simulink model "x_loop"  (Simulink 8.2)
settings: Solver=ode45  StartTime=0.0  StopTime=50  RelTol=1e-3
undefined symbols (not defined in the file): P
settings Model: Creator=paul  LastModifiedBy=paul
settings DataIOCC: SignalLoggingSaveFormat=Dataset
settings OptimizationCC: ExpressionDepthLimit=128
settings DebuggingCC: FcnCallInpInsideContextMsg=EnableAllAsError  StateNameClashWarn=none
settings GRTTargetCC: CombineOutputUpdateFcns=on  GRTInterface=off
settings ConfigurationSet: Description=SimMechanics 2G

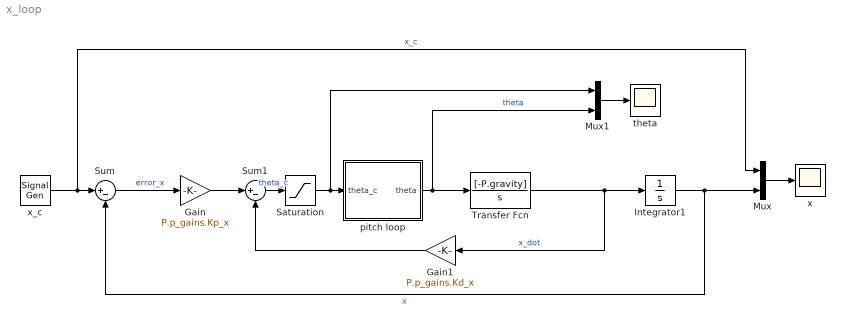
== system x_loop ==
  Gain : Gain  Gain=P.p_gains.Kp_x
  Gain1 : Gain  Gain=P.p_gains.Kd_x
  Integrator1 : Integrator
  Mux : Mux  Inputs=2
  Mux1 : Mux  Inputs=2
  Saturation : Saturate  UpperLimit=P.pitch_c_max  LowerLimit=-P.pitch_c_max
  Sum : Sum  Inputs=|+-
  Sum1 : Sum  Inputs=|+-
  Transfer Fcn : TransferFcn  Numerator=[-P.gravity]  Denominator=[1 0]
  pitch loop : Subsystem
  theta : Scope
      settings: YMin=-50  YMax=750
  x : Scope
      settings: TimeRange=50  YMin=-0.4  YMax=0.3
  x_c : SignalGenerator  WaveForm=square  Amplitude=0.25  Frequency=.05
  wires:
  Mux/1 -> x/1
  x_c/1 -> Mux/1, Sum/1  "x_c"
  Integrator1/1 -> Mux/2, Sum/2  "x"
  Gain1/1 -> Sum1/2
  Sum/1 -> Gain/1  "error_x"
  Gain/1 -> Sum1/1
  Mux1/1 -> theta/1
  Transfer Fcn/1 -> Integrator1/1, Gain1/1  "x_dot"
  Sum1/1 -> Saturation/1  "theta_c"
  pitch loop/1(theta) -> Transfer Fcn/1, Mux1/2  "theta"
  Saturation/1 -> pitch loop/1(theta_c), Mux1/1

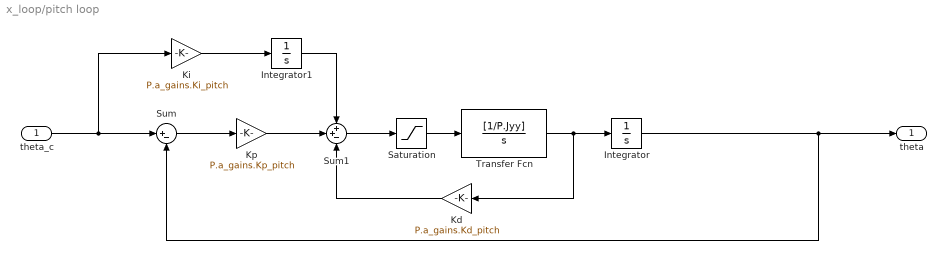
== system x_loop/pitch loop ==
  theta_c : Inport
  Integrator : Integrator
  Integrator1 : Integrator
  Kd : Gain  Gain=P.a_gains.Kd_pitch
  Ki : Gain  Gain=P.a_gains.Ki_pitch
  Kp : Gain  Gain=P.a_gains.Kp_pitch
  Saturation : Saturate
  Sum : Sum  Inputs=|+-
  Sum1 : Sum  Inputs=++-
  Transfer Fcn : TransferFcn  Numerator=[1/P.Jyy]  Denominator=[1 0]
  theta : Outport
  wires:
  Kp/1 -> Sum1/2
  theta_c/1 -> Ki/1, Sum/1
  Transfer Fcn/1 -> Kd/1, Integrator/1
  Integrator/1 -> Sum/2, theta/1
  Saturation/1 -> Transfer Fcn/1
  Ki/1 -> Integrator1/1
  Sum1/1 -> Saturation/1
  Kd/1 -> Sum1/3
  Integrator1/1 -> Sum1/1
  Sum/1 -> Kp/1
